simulink model "Movimiento_traslacional_simulink"  (R2023b)
settings: Solver=VariableStepAuto  StartTime=0.0  StopTime=10.0  RelTol=1e-3
values from neighbouring files (symbols this model uses):
  b1 = 1000    [Movimiento_traslacional.m]    (also in ParametrosP3.m)
  f = 0    [Movimiento_traslacional.m]    (also in ParametrosP3.m)
  k1 = 16182    [Movimiento_traslacional.m]    (also in ParametrosP3.m)
  k2 = 19000    [Movimiento_traslacional.m]    (also in ParametrosP3.m)
  m1 = 290    [Movimiento_traslacional.m]    (also in ParametrosP3.m)
  m2 = 59    [Movimiento_traslacional.m]    (also in ParametrosP3.m)
settings Model: Creator=52466
settings OptimizationCC: ReuseModelBlockBuffer=off

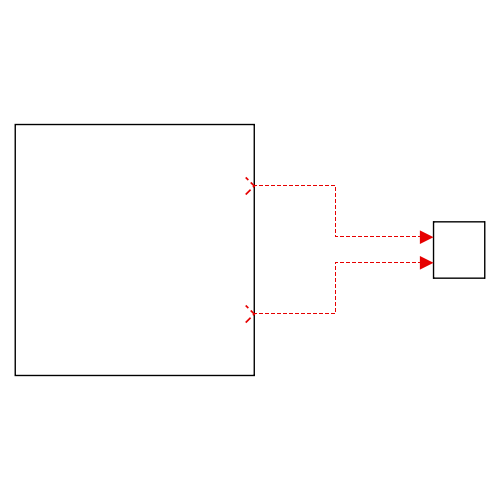
[thumbnail: Simulink's stored preview of the top-level diagram]
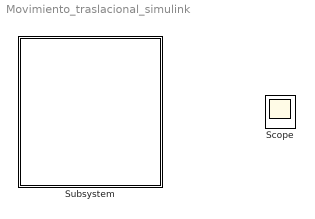
== system Movimiento_traslacional_simulink ==
  Scope : Scope  NumInputPorts=2
  Subsystem : Subsystem
  wires:
  ? -> Scope/1
  ? -> Scope/2

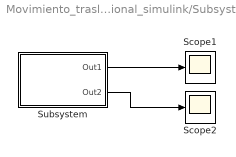
== system Movimiento_traslacional_simulink/Subsystem ==
  Scope1 : Scope
  Scope2 : Scope
  Subsystem : Subsystem
  wires:
  Subsystem/2(Out2) -> Scope2/1
  Subsystem/1(Out1) -> Scope1/1

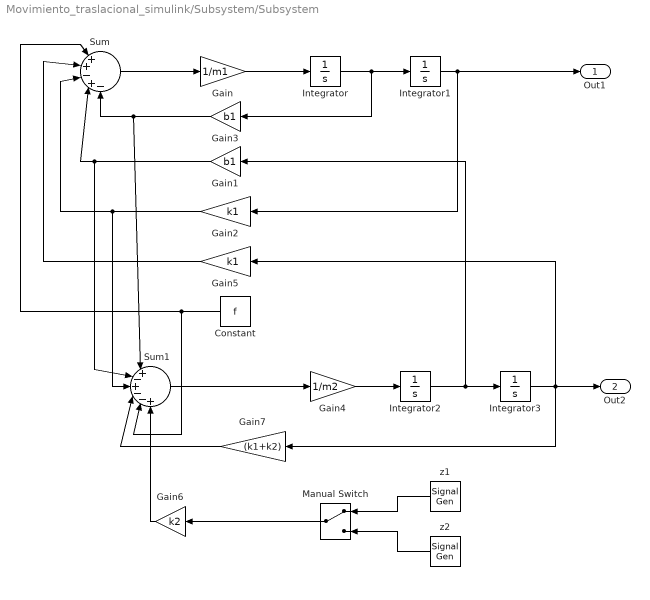
== system Movimiento_traslacional_simulink/Subsystem/Subsystem ==
  Constant : Constant  Value=f
  Gain : Gain  Gain=1/m1
  Gain1 : Gain  Gain=b1
  Gain2 : Gain  Gain=k1
  Gain3 : Gain  Gain=b1
  Gain4 : Gain  Gain=1/m2
  Gain5 : Gain  Gain=k1
  Gain6 : Gain  Gain=k2
  Gain7 : Gain  Gain=(k1+k2)
  Integrator{,1..3} (4 alike) : Integrator
  Manual Switch : ManualSwitch
  Sum : Sum  Inputs=|++-+-
  Sum1 : Sum  Inputs=|+-+--+
  z1 : SignalGenerator  Amplitude=0.05  Frequency=0.5*pi  Units=rad/sec
  z2 : SignalGenerator  Amplitude=0.05  Frequency=20*pi  Units=rad/sec
  Out1 : Outport
  Out2 : Outport  Port=2
  wires:
  Manual Switch/1 -> Gain6/1
  z2/1 -> Manual Switch/2
  z1/1 -> Manual Switch/1
  Gain6/1 -> Sum1/6
  Integrator/1 -> Integrator1/1, Gain3/1
  Gain/1 -> Integrator/1
  Gain2/1 -> Sum1/3, Sum/3
  Integrator3/1 -> Gain5/1, Gain7/1, Out2/1
  Integrator2/1 -> Integrator3/1, Gain1/1
  Sum/1 -> Gain/1
  Constant/1 -> Sum/1, Sum1/5
  Gain4/1 -> Integrator2/1
  Gain5/1 -> Sum/2
  Gain1/1 -> Sum1/2, Sum/4
  Sum1/1 -> Gain4/1
  Gain7/1 -> Sum1/4
  Gain3/1 -> Sum1/1, Sum/5
  Integrator1/1 -> Gain2/1, Out1/1
